simulink library "BSCU_lib"  (R2016a)
settings: Solver=ode45  StartTime=0.0  StopTime=10.0  RelTol=1e-3
settings Model: Creator=jliu29  LastModifiedBy=jliu29
settings DataIOCC: LimitDataPoints=on
settings DebuggingCC: AllowSymbolicDim=off

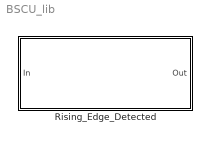
== system BSCU_lib ==
  Rising_Edge_Detected : Subsystem

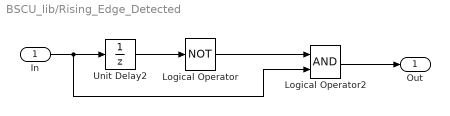
== system BSCU_lib/Rising_Edge_Detected ==
  In : Inport
  Logical Operator : Logic  Operator=NOT  AllPortsSameDT=off  OutDataTypeStr=boolean
  Logical Operator2 : Logic  AllPortsSameDT=off  OutDataTypeStr=boolean
  Unit Delay2 : UnitDelay  SampleTime=-1
      settings: AttributesFormatString=<Init = %<InitialCondition>>
  Out : Outport
  wires:
  Logical Operator2/1 -> Out/1
  In/1 -> Logical Operator2/2, Unit Delay2/1
  Unit Delay2/1 -> Logical Operator/1
  Logical Operator/1 -> Logical Operator2/1
